simulink model "Magman_plain"  (R2016b)
settings: Solver=VariableStepAuto  StartTime=0.0  StopTime=10.0  RelTol=1e-3
values from neighbouring files (symbols this model uses):
  a = 5.713e-09    [LQI_script.m]    (also in PID_script.m = 4.367e-09; fminsim.m = block.InputPort(3).Data; model_generation.m = 4.367e-09)
  b = 0.000324    [LQI_script.m]    (also in PID_script.m = 0.0002827; fminsim.m = block.InputPort(4).Data; model_generation.m = 0.0002827)
  m = 56.3/1000    (= 0.0563)    [LQI_script.m]    (also in PID_script.m; model_generation.m)
  mu = 0.04    [LQI_script.m]    (also in PID_script.m)
  pos_var = 5e-09    [LQI_script.m]    (also in PID_script.m)
  x00 = linpos-0.013    (= 0.04955)    [LQI_script.m]    (also in PID_script.m = 0.03)
  x1 = 0.02525    [LQI_script.m]    (also in PID_script.m; fminsim.m = block.InputPort(5).Data; model_generation.m)
  x2 = 0.05    [LQI_script.m]    (also in PID_script.m; fminsim.m = block.InputPort(6).Data; model_generation.m)
  x3 = 0.0751    [LQI_script.m]    (also in PID_script.m; fminsim.m = block.InputPort(7).Data; model_generation.m)
  x4 = 0.103    [LQI_script.m]    (also in PID_script.m; fminsim.m = block.InputPort(8).Data; model_generation.m)
libraries: dspsrcs4 x1
settings Model: Creator=Andres  LastModifiedBy=Andres

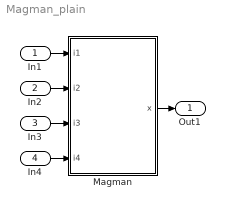
== system Magman_plain ==
  In1 : Inport
  In2 : Inport  Port=2
  In3 : Inport  Port=3
  In4 : Inport  Port=4
  Magman : Subsystem
  Out1 : Outport
  wires:
  In1/1 -> Magman/1(i1)
  In2/1 -> Magman/2(i2)
  In3/1 -> Magman/3(i3)
  In4/1 -> Magman/4(i4)
  Magman/1(x) -> Out1/1

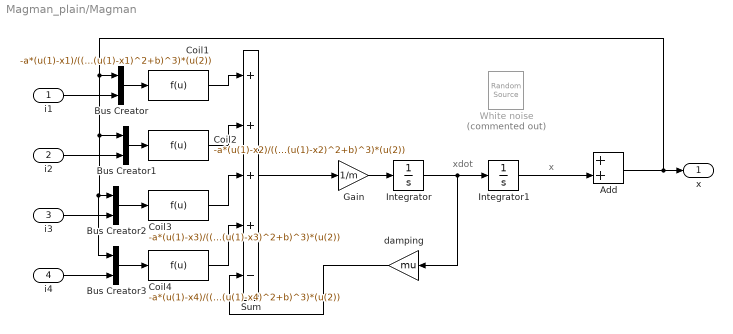
== system Magman_plain/Magman ==
  note: x
  note: xdot
  i1 : Inport
  i2 : Inport  Port=2
  i3 : Inport  Port=3
  i4 : Inport  Port=4
  Add : Sum
  Bus Creator{,1..3} (4 alike) : BusCreator  Inputs=2
  Coil1 : Fcn  Expr=-a*(u(1)-x1)/(((u(1)-x1)^2+b)^3)*(u(2))
  Coil2 : Fcn  Expr=-a*(u(1)-x2)/(((u(1)-x2)^2+b)^3)*(u(2))
  Coil3 : Fcn  Expr=-a*(u(1)-x3)/(((u(1)-x3)^2+b)^3)*(u(2))
  Coil4 : Fcn  Expr=-a*(u(1)-x4)/(((u(1)-x4)^2+b)^3)*(u(2))
  Gain : Gain  Gain=1/m
  Integrator : Integrator  ContinuousStateAttributes='xdot'
  Integrator1 : Integrator  InitialCondition=x00  ContinuousStateAttributes='x'
  Sum : Sum  Inputs=++++-
  White noise : dspsrcs4/Random Source  Commented=on  SrcType=Gaussian  NormMethod=Ziggurat  CltLength=12  MinVal=0  MaxVal=1  MeanVal=0  VarVal=2*pos_var  RepMode=Not repeatable  rawSeed=1  IsInherit=off  SampMode=Discrete  SampTime=h  SampFrame=1  DataType=Double  OutComplex=Real  OutputFrames=off
  damping : Gain  Gain=mu
  x : Outport
  wires:
  Bus Creator/1 -> Coil1/1
  Coil2/1 -> Sum/2
  i1/1 -> Bus Creator/2
  Integrator1/1 -> Add/2
  Integrator/1 -> damping/1, Integrator1/1
  Bus Creator2/1 -> Coil3/1
  i4/1 -> Bus Creator3/2
  Bus Creator3/1 -> Coil4/1
  Coil1/1 -> Sum/1
  i2/1 -> Bus Creator1/2
  i3/1 -> Bus Creator2/2
  Gain/1 -> Integrator/1
  Coil4/1 -> Sum/4
  Coil3/1 -> Sum/3
  Bus Creator1/1 -> Coil2/1
  damping/1 -> Sum/5
  Add/1 -> Bus Creator3/1, Bus Creator2/1, Bus Creator1/1, Bus Creator/1, x/1
  Sum/1 -> Gain/1
